simulink model "probe"  (R2013b)
settings: Solver=ode45  StartTime=0.0  StopTime=10.0  MaxStep=0.002  MinStep=0.001  RelTol=1e-3
undefined symbols (not defined in the file or in its folder): i
settings Model: Creator=user  LastModifiedBy=user

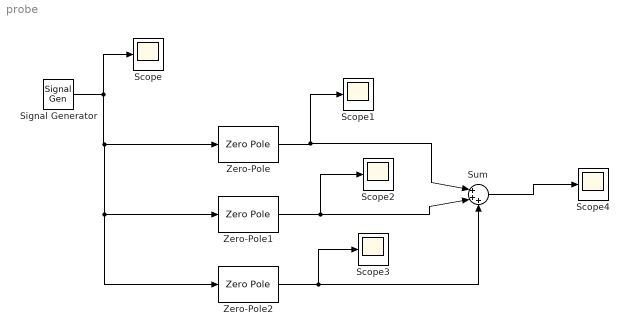
== system probe ==
  Scope{,1..4} (5 alike) : Scope
      Scope2 settings: SaveName=ScopeData2
      Scope3 settings: SaveName=ScopeData3
      Scope4 settings: SaveName=ScopeData4
  Signal Generator : SignalGenerator  WaveForm=sawtooth  Frequency=25  Units=rad/sec
  Sum : Sum  Inputs=|+++
  Zero-Pole : ZeroPole  Poles=[-0.005*25+i*25*0.9999875 , -0.005*25-i*25*0.9999875]
  Zero-Pole1 : ZeroPole  Poles=[-0.005*25*2+i*25*2*0.9999875 , -0.005*2*25-i*25*2*0.9999875]
  Zero-Pole2 : ZeroPole  Poles=[-0.005*25*3+i*25*3*0.9999875 , -0.005*3*25-i*25*3*0.9999875]
  wires:
  Zero-Pole/1 -> Sum/1, Scope1/1
  Zero-Pole1/1 -> Sum/2, Scope2/1
  Zero-Pole2/1 -> Sum/3, Scope3/1
  Sum/1 -> Scope4/1
  Signal Generator/1 -> Zero-Pole2/1, Zero-Pole1/1, Zero-Pole/1, Scope/1
